simulink model "BLEMeshDiscreteEventSimulationModel"  (R2021a)
settings: Solver=VariableStepDiscrete  StartTime=0.0  StopTime=3  MaxStep=inf  RelTol=1e-3
PostLoadFcn:
  | load('bleMeshBusObjects.mat');
  | load('bleMeshDESNodePositions.mat');
  | ModelName = bdroot;
  | helperBLEMeshAssignNodeIDs(ModelName);
  | NumberOfNodes = numel(helperBLEMeshGetNodeNamesList(ModelName));
  | % Statistics
  | opcode = 0; % For creating the table
  | helperBLEMeshUpdateStatistics(opcode);
  | meshNetworkGraph = helperBLEMeshVisualizeNetwork();
InitFcn:
  | load('bleMeshBusObjects.mat');
  | load('bleMeshDESNodePositions.mat');
  | ModelName = bdroot;
  | helperBLEMeshAssignNodeIDs(ModelName);
  | NumberOfNodes = numel(helperBLEMeshGetNodeNamesList(ModelName));
  | % Statistics
  | opcode = 0; % For creating the table
  | helperBLEMeshUpdateStatistics(opcode);
  | meshNetworkGraph = helperBLEMeshVisualizeNetwork();
  | rng('default');
StartFcn:
  | if enableVisualization == 1
  | meshNetworkGraph.createNetwork();
  | end
StopFcn:
  | % Sort statisticsAtEachNode table
  | list = statisticsAtEachNode.Properties.RowNames;
  | nodeNum = cellfun(@(x)sscanf(x,'Node%d'), list);
  | [~,sortIdx] = sort(nodeNum);
  | statisticsAtEachNode = statisticsAtEachNode(sortIdx, :);
  | 
  | % Fill node statisticsAtEachNode in a cell array as input to visualization object
  | nodeStatistics = cell(1, NumberOfNodes);
  | for idx = 1:NumberOfNodes
  |     stats = {
  |         'Node Type', statisticsAtEachNode{idx, 'NodeType'}, ...
  |         'PHYTransmittedSignals', statisticsAtEachNode{idx, 'PHYTransmittedSignals'}, ...
  |         'PHYReceivedSignals', statisticsAtEachNode{idx, 'PHYReceivedSignals'}, ...
  |         'TotalCollisions', statisticsAtEachNode{idx, 'TotalCollisions'}, ...
  |         'LinkLayerTransmittedMsgs', statisticsAtEachNode{idx, 'LinkLayerTransmittedMsgs'}, ...
  |         'LinkLayerReceivedMsgs', statisticsAtEachNode{idx, 'LinkLayerReceivedMsgs'}, ...
  |         'CRCFailedMsgs', statisticsAtEachNode{idx, 'CRCFailedMsgs'}, ...
  |         'NetworkLayerTransmittedMsgs', statisticsAtEachNode{idx, 'NetworkLayerTransmittedMsgs'}, ...
  |         'NetworkLayerReceivedMsgs', statisticsAtEachNode{idx, 'NetworkLayerReceivedMsgs'}, ...
  |         'ReceivedApplicationMsgs', statisticsAtEachNode{idx, 'ReceivedApplicationMsgs'}, ...
  |         'NetworkLayerRelayedMsgs', statisticsAtEachNode{idx, 'NetworkLayerRelayedMsgs'}, ...
  |         'NetworkLayerDroppedMsgs', statisticsAtEachNode{idx, 'NetworkLayerDroppedMsgs'}};
  |     nodeStatistics{idx} = stats;
  | end
  | % Update statisticsAtEachNode in visualization object
  | if enableVisualization == 1
  | meshNetworkGraph.updateNodeStatistics(nodeStatistics);
  | end
  | % Calculate PDR of network
  | PDR = sum(statisticsAtEachNode.ReceivedApplicationMsgs) / sum(statisticsAtEachNode.NetworkLayerTransmittedMsgs);
  | fprintf('Network PDR is: %f\n', round(PDR, 4));
values from neighbouring files (symbols this model uses):
  bleMeshDESNodePositions = [0 2 4 6 8 10 12 14 16 18 20 22 ... (300 elements, 100x3)]    [bleMeshDESNodePositions.mat]    (also in bleMeshDESNodePositions19.mat = [5.030833333 8.024583333 13.395 16.32708333 22.90125 22.9012; bleMeshDESNodePositions38.mat = [2.7 5.45 5.825 10.65 13.5 13.875 18.65 21.4 18.55 2.7 5.45 ; bleMeshDESNodePositions51.mat = [2.45 5.4 2.45 5.4 5.75 10.375 13.3 10.375 13.3 13.75 18.75 ; bleMeshDESNodePositions68.mat = [0 2 4 6 8 10 12 14 16 18 0 2 ... (300 elements, 100x3)])
undefined symbols (not defined in the file or in its folder): m
libraries: BLEMeshLib x10
PostSaveFcn:
  | load('bleMeshBusObjects.mat');
  | load('bleMeshDESNodePositions.mat');
  | ModelName = bdroot;
  | helperBLEMeshAssignNodeIDs(ModelName);
  | NumberOfNodes = numel(helperBLEMeshGetNodeNamesList(ModelName));
  | % Statistics
  | opcode = 0; % For creating the table
  | helperBLEMeshUpdateStatistics(opcode);
  | meshNetworkGraph = helperBLEMeshVisualizeNetwork();
settings Model: Creator=The MathWorks, Inc.  LastModifiedBy=qcnguyen
settings SolverCC: AlgebraicLoopSolver=TrustRegion
settings DebuggingCC: SFMachineParentedDataDiag=warning

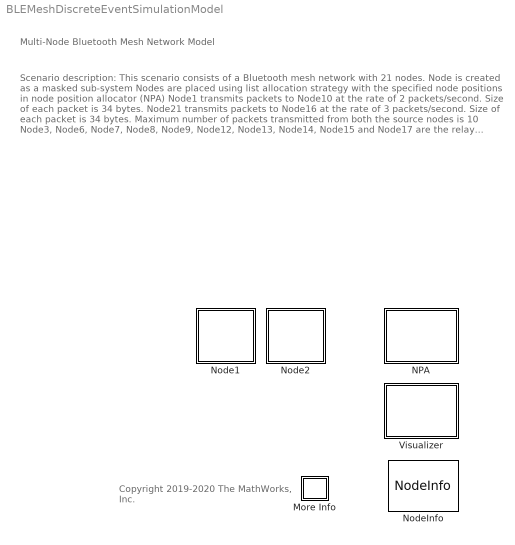
== system BLEMeshDiscreteEventSimulationModel ==
  note: Copyright 2019-2020 The MathWorks, Inc.
  note: Multi-Node Bluetooth Mesh Network Model
  note: Scenario description:
      | This scenario consists of a Bluetooth mesh network with 21 nodes. Node is created as a masked sub-system
      | Nodes are placed using list allocation strategy with the specified node positions in node position allocator (NPA)
      | Node1 transmits packets to Node10 at the rate of 2 packets/second. Size of each packet is 34 bytes.
      | Node21 transmits packets to Node16 at the rate of 3 packets/second. Size of each packet is 34 bytes.
      | Maximum number of packets transmitted from both the source nodes is 10
      | Node3, Node6, Node7, Node8, Node9, Node12, Node13, Node14, Node15 and Node17 are the relay nodes
      | Simulation time is set to 3 seconds
      | Each node contains:
      | Bluetooth mesh packet generator and receiver (mesh packet includes model, access and transport layer encoding and decoding)
      | Bluetooth mesh network layer
      | BLE link layer
      | BLE PHY Tx and Rx including interference modeling
      | Channel model
      | Nodes communicate using shared channel
      | NPA sets location of all the nodes at the start of simulation
      | Visualizer block visualizes the mesh network scenario
  More Info : Subsystem
      settings: OpenFcn=showExample('bluetooth/BLEMeshDiscreteEventSimulationExample')
      mask Display: disp('?')
  NPA : Subsystem  Tag=a  Priority=100  mask(NPA){numOfNodes=NumberOfNodes, allocationType=List Position Allocation, delta=25, direction=X, initX=0, initY=0, GridDeltaX=3, GridDeltaY=3, GridWidth=10, listName=bleMeshDESNodePositions}
      mask prompts: numOfNodes "Number of nodes:"; allocationType "Type of position allocation:"; initX "Initial X:"; initY "Initial Y:"; GridDeltaX "Delta X:"; GridDeltaY "Delta Y:"; GridWidth "Width:"; listName "Node positions:"
      mask help:
      | This block allocates node positions using three different allocation strategies –
      |
      | Linear position allocation: Places nodes uniformly in a vertical or a horizontal straight line.
      |
      | Grid position allocation: Places nodes in a grid specified by the grid properties. These properties include - direction to assign node position in the grid, initial X-Y coordinates denoting the starting location of grid, spacing in X and Y direction between successive nodes, and the number of nodes placed in a vertical or a horizontal line.
      |
      | List position allocation: Places nodes specified by a list. The list is in the form of a N-by-3 matrix, where N represents the total number of nodes and each row vector of the matrix denotes the x, y, and z coordinates of a node.
      |
      | Each of the above node position allocation strategy follows this format to specify the name of each node – <Node><n>. For example, in a network consisting of two nodes, the names of nodes can be (Node1, Node2) or (Node2, Node1).
      mask init:
      | % Visualization object
      | coder.extrinsic('assignin', 'evalin');
      | meshNetworkGraph = evalin('base', 'meshNetworkGraph');
      | 
      | % Get initial node positions by calling node position allocation strategies
      | positions = zeros(numOfNodes, 3);
      | 
      | % Linear allocation
      | if (allocationType == 1)
      |     % Allocate positions in a line with constant distance between nodes.
      |     count = 0;
      |     for i = 1:numOfNodes
      |         switch(direction)
      |             % Allocate positions in a horizontal line
      |             case 1
      |                 positions(i, 1) = initX+ delta*count;
      |                 positions(i, 2) = initY;
      |                 positions(i, 3) = 0;
      |                 % Allocate positions in a vertical line
      |             case 2
      |                 positions(i, 1) = initX;
      |                 positions(i, 2) = initY+ delta*count;
      |                 positions(i, 3)= 0;
      |         end
      |         count = count + 1;
      |     end
      |     
      | % Grid allocation 
      | elseif (allocationType == 2)
      |     for i = 1:(numOfNodes)
      |         switch(direction)
      |             case 1 % Arrange nodes row by row
      |                 positions(i, 1) = initX + GridDeltaX*(mod(i-1, GridWidth));
      |                 positions(i, 2) = initY + GridDeltaY*(floor((i-1)/GridWidth));
      |                 positions(i, 3) = 0;
      |             case 2 % Arrange nodes column by column
      |                 positions(i, 1) = initX + GridDeltaX*(floor(i-1/GridWidth));
      |                 positions(i, 2) = initY + GridDeltaY*(mod(i-1, GridWidth));
      |                 positions(i, 3) = 0;
      |         end
      |     end
      |         
      | % List allocation    
      | elseif (allocationType == 3)
      |     % Allocates node positions from a list specified by the user.
      |     positions = listName(1:(numOfNodes), :, :);
      | end
      | 
      | % Set the positions of nodes
      | for i = 1:numOfNodes
      |     % Get the block which contains matching node id as a parameter
      |     blockName = find_system(bdroot,'NodeID',num2str(i));
      |     posID = str2num(blockName{1}(strlength([bdroot '/Node'])+1:end));
      |     try
      |         % Convert position from number to string
      |         b = num2str(['[' [num2str(positions(posID, :)) ']']]);
      |         % Assign new position to a node subsystem
      |         set_param(blockName{1},'NodePosition', b);
      |     catch
      |     end
      | end
      | 
      | positions = positions(:,1:2);
      | 
      | % Update configuration
      | meshNetworkGraph.NumberOfNodes = numOfNodes;
      | meshNetworkGraph.NodePositionType = 'UserInput';
      | meshNetworkGraph.Positions = positions;
      | %meshNetworkGraph.VicinityRange = 25;
      | meshNetworkGraph.Title = 'Bluetooth Mesh Network';
      | 
      | assignin('base', 'meshNetworkGraph', meshNetworkGraph);
      mask TypeOptions allocationType: Linear Position Allocation | Grid Position Allocation | List Position Allocation
      mask Callback allocationType:
      | % Get allocation type selected by user
      | maskStr = get_param(gcb,'allocationType');
      | % Set mask parameters visibilities based on allocation type
      | if strcmp(maskStr,'Linear Position Allocation')
      |     set_param(gcb,'MaskVisibilities',{'on','on','on','on','on','on','off','off','off','off'});
      | elseif strcmp(maskStr,'List Position Allocation')
      |     set_param(gcb,'MaskVisibilities',{'on','on','off','off','off','off','off','off','off','on'});
      | elseif strcmp(maskStr,'Grid Position Allocation')
      |     set_param(gcb,'MaskVisibilities',{'on','on','off','on','on','on','on','on','on','off'});
      | end
      | % Clear variables
      | clear maskStr;
      mask TypeOptions direction: X | Y
      mask Display: disp('NPA');
  Node1 : Subsystem  mask{NodePosition=[2.45        1.65           0], NodeID=1}
      mask prompts: NodePosition "Node position:"; NodeID "Node id:"
      mask init:
      | global NodeInfo
      | ElementAddress = hex2dec(reshape(dec2hex(NodeID, 4), 2, [])');
      | NodeInfo(NodeID).NodeID = NodeID;
      | NodeInfo(NodeID).ElementAddress = ElementAddress;
      mask DialogControl DescGroupVar Prompt: Bluetooth device
      mask DialogControl DescTextVar Prompt: Bluetooth mesh device communicates over GAP bearer including:  Application layer, Network layer, Link layer and Physical layer
      mask Display: disp(['Bluetooth' newline 'Node']);
  Node2 : Subsystem  mask{NodePosition=[5.4        1.65           0], NodeID=2}
      mask prompts: NodePosition "Node position:"; NodeID "Node id:"
      mask init:
      | global NodeInfo
      | ElementAddress = hex2dec(reshape(dec2hex(NodeID, 4), 2, [])');
      | NodeInfo(NodeID).NodeID = NodeID;
      | NodeInfo(NodeID).ElementAddress = ElementAddress;
      mask DialogControl DescGroupVar Prompt: Bluetooth device
      mask DialogControl DescTextVar Prompt: Bluetooth mesh device communicates over GAP bearer including:  Application layer, Network layer, Link layer and Physical layer
      mask Display: disp(['Bluetooth' newline 'Node']);
  NodeInfo : DataStoreMemory  DataStoreName=NodeInfo  ReadBeforeWriteMsg=warning  WriteAfterWriteMsg=warning  WriteAfterReadMsg=warning  ShowAdditionalParam=off  OutDataTypeStr=Bus: NodeInfo  Dimensions=NumberOfNodes
      mask DialogControl DescGroupVar Prompt: NodeInfo
      mask DialogControl DescTextVar Prompt: This block is used to store and share node-related information such as NodeID and ElementAddress. There are no configuration options for this block.
  Visualizer : Subsystem  Tag=a  Priority=100  mask(Subsystem){enableVisualization=on}
      mask prompts: enableVisualization "Enable Visualization"
      mask init:
      | % Skip codegen
      | coder.extrinsic('assignin', 'evalin', 'get_param');
      | assignin('base', 'enableVisualization', enableVisualization);
      | % If visualization is enabled update the configuration in visualization
      | % object
      | if (enableVisualization == 1)
      |     meshNetworkGraph = evalin('base', 'meshNetworkGraph');
      |     NumberOfNodes = evalin('base', 'NumberOfNodes');
      |     % Get srcDstPairs and relayNodes from assigned configuration
      |     srcDstPairs = zeros(1, 0);
      |     relayNodes = zeros(1, 0);
      |     srcDstPairsIdx = 1;
      |     relayIdx = 1;
      |     for i = 1:NumberOfNodes
      |         appState = get_param([bdroot '/Node' num2str(i) '/AppDES'], 'ApplicationState');
      |         if strcmp(appState, '0') == false
      |             destName = get_param([bdroot '/Node' num2str(i) '/AppDES'], 'DestinationNode');
      |             %str = split(destName, 'e');
      |             srcDstPairs(srcDstPairsIdx, 1) = i;
      |             srcDstPairs(srcDstPairsIdx, 2) = str2double(destName);
      |             %srcDstPairs(srcDstPairsIdx, 2) = str2double(str{2});
      |             srcDstPairsIdx = srcDstPairsIdx + 1;
      |         end
      |         relay = get_param([bdroot '/Node' num2str(i) '/Network layer'], 'Relay');
      |         if strcmp(relay, 'Off') == false
      |             relayNodes(relayIdx) = i;
      |             relayIdx = relayIdx + 1;
      |         end
      |     end
      |     meshNetworkGraph.NumberOfNodes = NumberOfNodes;
      |     meshNetworkGraph.SrcDstPairs = srcDstPairs;
      |     nodeStates = zeros(1, NumberOfNodes);
      |     for i=1:NumberOfNodes
      |         % Relay node
      |         if any(i == relayNodes)
      |             nodeStates(i) = 2;
      |             % End node
      |         else
      |             nodeStates(i) = 1;
      |         end
      |     end
      |     meshNetworkGraph.NodeState = nodeStates;
      |     meshNetworkGraph.DisplayProgressBar = false;
      |     assignin('base', 'meshNetworkGraph', meshNetworkGraph);
      | end
      mask DialogControl DescGroupVar Prompt: Visualizer
      mask DialogControl DescTextVar Prompt: Visualizes Bluetooth mesh network based on the given configuration
      mask Display: disp('Visualizer');

== system BLEMeshDiscreteEventSimulationModel/More Info ==

== system BLEMeshDiscreteEventSimulationModel/NPA ==

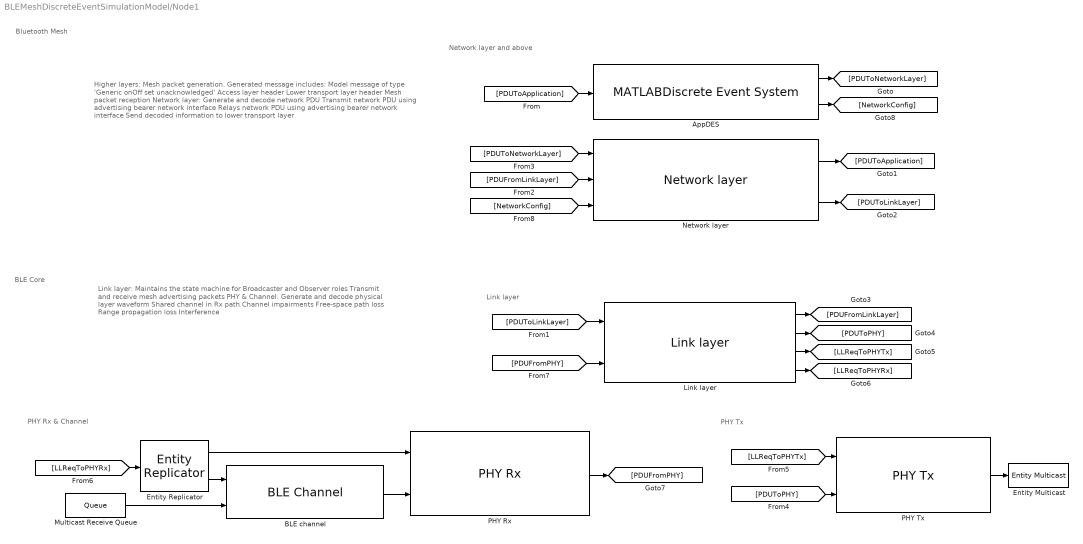
== system BLEMeshDiscreteEventSimulationModel/Node1 ==
  note: Network layer and above
  note: Link layer
  note: Link layer:
      | Maintains the state machine for Broadcaster and Observer roles
      | Transmit and receive mesh advertising packets
      |
      | PHY & Channel:
      | Generate and decode physical layer waveform
      | Shared channel in Rx path
      | Channel impairments
      | Free-space path loss
      | Range propagation loss
      | Interference
  note: BLE Core
  note: Bluetooth Mesh
  note: PHY Rx & Channel
  note: PHY Tx
  note: Higher layers:
      | Mesh packet generation. Generated message includes:
      | Model message of type 'Generic onOff set unacknowledged'
      | Access layer header
      | Lower transport layer header
      | Mesh packet reception
      |
      | Network layer:
      | Generate and decode network PDU
      | Transmit network PDU using advertising bearer network interface
      | Relays network PDU using advertising bearer network interface
      | Send decoded information to lower transport layer
  AppDES : MATLABDiscreteEventSystem  InputPortMessageModes=m  OutputPortMessageModes=m,m  System=AppDES  NodeID=1  DestinationNode=1  ApplicationState=0  TTL=127  SourceRate=1  TotalPackets=1  SimulateUsing=Code generation
      mask Type: AppDES
      mask Display:
      | disp('AppDES');
      | port_label('input',1,'transportPDUIn');
      | port_label('output',1,'transportPDUOut');
      | port_label('output',2,'networkConfig');
  BLE channel : BLEMeshLib/BLE Channel  RangePropagationLoss=On  FSPLModel=On  RxRange=7  NodePosition=NodePosition  NodeID=NodeID  SimulateUsing=Code generation
  Entity Multicast : EntityMulticast  InputPortMessageModes=m  MulticastTag=channel
  Entity Replicator : EntityReplicator  InputPortMessageModes=m  OutputPortMessageModes=m,m
  Link layer : BLEMeshLib/Link layer  RandomAdvertising=On  AdvertisingInterval=20  ScanInterval=30  NodeID=NodeID  SimulateUsing=Code generation  mask(helperBLEMeshLinkLayerDES){}
  Multicast Receive Queue : Queue  OutputPortMessageModes=m  EntityArrivalSource=Multicast  MulticastTag=channel
  Network layer : BLEMeshLib/Network layer  Relay=Off  ElementAddresses=ElementAddress  NetworkTransmitCount=3  NetworkTransmitInterval=30  RelayRetransmitCount=3  RelayRetransmitInterval=30  NodeID=NodeID  SimulateUsing=Code generation
  PHY Rx : BLEMeshLib/PHY Rx  NoiseFigure=0  NodeID=NodeID  SimulateUsing=Interpreted execution
  PHY Tx : BLEMeshLib/PHY Tx  TxPower=0  NodePosition=NodePosition  NodeID=NodeID  SimulateUsing=Interpreted execution
  wires:
  Link layer/4 -> [LLReqToPHYRx]
  Link layer/2 -> [PDUToPHY]
  Link layer/3 -> [LLReqToPHYTx]
  Link layer/1 -> [PDUFromLinkLayer]
  [PDUToNetworkLayer] -> Network layer/1
  Network layer/1 -> [PDUToApplication]
  [PDUFromLinkLayer] -> Network layer/2
  Entity Replicator/1 -> PHY Rx/1
  PHY Rx/1 -> [PDUFromPHY]
  BLE channel/1 -> PHY Rx/2
  PHY Tx/1 -> Entity Multicast/1
  [LLReqToPHYRx] -> Entity Replicator/1
  Multicast Receive Queue/1 -> BLE channel/2
  Entity Replicator/2 -> BLE channel/1
  [LLReqToPHYTx] -> PHY Tx/1
  [PDUToPHY] -> PHY Tx/2
  Network layer/2 -> [PDUToLinkLayer]
  [PDUToLinkLayer] -> Link layer/1
  [PDUFromPHY] -> Link layer/2
  AppDES/1 -> [PDUToNetworkLayer]
  [PDUToApplication] -> AppDES/1
  [NetworkConfig] -> Network layer/3
  AppDES/2 -> [NetworkConfig]

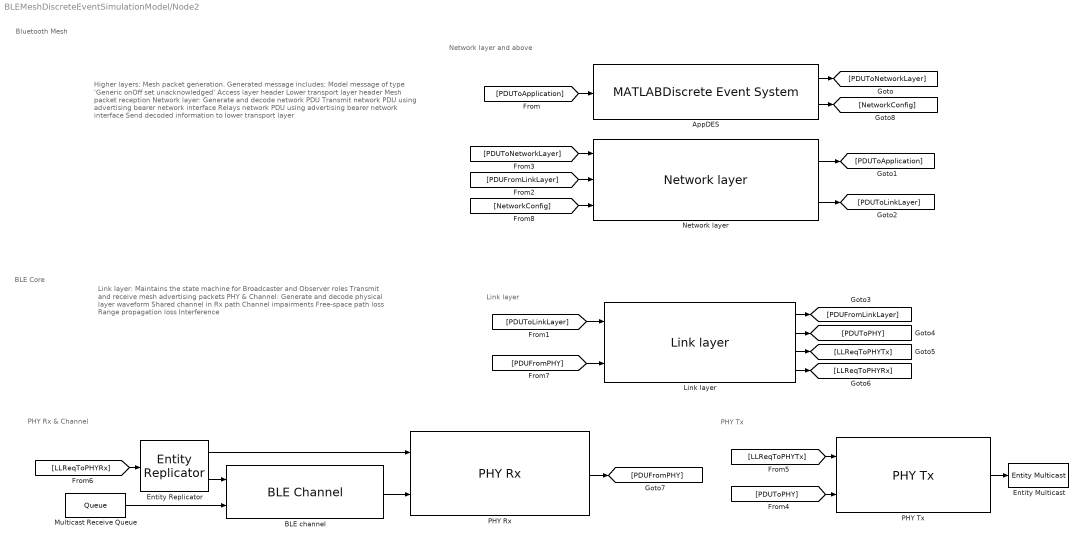
== system BLEMeshDiscreteEventSimulationModel/Node2 ==
  note: Network layer and above
  note: Link layer
  note: Link layer:
      | Maintains the state machine for Broadcaster and Observer roles
      | Transmit and receive mesh advertising packets
      |
      | PHY & Channel:
      | Generate and decode physical layer waveform
      | Shared channel in Rx path
      | Channel impairments
      | Free-space path loss
      | Range propagation loss
      | Interference
  note: BLE Core
  note: Bluetooth Mesh
  note: PHY Rx & Channel
  note: PHY Tx
  note: Higher layers:
      | Mesh packet generation. Generated message includes:
      | Model message of type 'Generic onOff set unacknowledged'
      | Access layer header
      | Lower transport layer header
      | Mesh packet reception
      |
      | Network layer:
      | Generate and decode network PDU
      | Transmit network PDU using advertising bearer network interface
      | Relays network PDU using advertising bearer network interface
      | Send decoded information to lower transport layer
  AppDES : MATLABDiscreteEventSystem  InputPortMessageModes=m  OutputPortMessageModes=m,m  System=AppDES  NodeID=2  DestinationNode=1  ApplicationState=0  TTL=127  SourceRate=1  TotalPackets=1  SimulateUsing=Code generation
      mask Type: AppDES
      mask Display:
      | disp('AppDES');
      | port_label('input',1,'transportPDUIn');
      | port_label('output',1,'transportPDUOut');
      | port_label('output',2,'networkConfig');
  BLE channel : BLEMeshLib/BLE Channel  RangePropagationLoss=On  FSPLModel=On  RxRange=6  NodePosition=NodePosition  NodeID=NodeID  SimulateUsing=Code generation
  Entity Multicast : EntityMulticast  InputPortMessageModes=m  MulticastTag=channel
  Entity Replicator : EntityReplicator  InputPortMessageModes=m  OutputPortMessageModes=m,m
  Link layer : BLEMeshLib/Link layer  RandomAdvertising=On  AdvertisingInterval=20  ScanInterval=30  NodeID=NodeID  SimulateUsing=Code generation  mask(helperBLEMeshLinkLayerDES){}
  Multicast Receive Queue : Queue  OutputPortMessageModes=m  EntityArrivalSource=Multicast  MulticastTag=channel
  Network layer : BLEMeshLib/Network layer  Relay=Off  ElementAddresses=ElementAddress  NetworkTransmitCount=3  NetworkTransmitInterval=30  RelayRetransmitCount=3  RelayRetransmitInterval=30  NodeID=NodeID  SimulateUsing=Code generation
  PHY Rx : BLEMeshLib/PHY Rx  NoiseFigure=0  NodeID=NodeID  SimulateUsing=Interpreted execution
  PHY Tx : BLEMeshLib/PHY Tx  TxPower=20  NodePosition=NodePosition  NodeID=NodeID  SimulateUsing=Interpreted execution
  wires:
  Link layer/4 -> [LLReqToPHYRx]
  Link layer/2 -> [PDUToPHY]
  Link layer/3 -> [LLReqToPHYTx]
  Link layer/1 -> [PDUFromLinkLayer]
  [PDUToNetworkLayer] -> Network layer/1
  Network layer/1 -> [PDUToApplication]
  [PDUFromLinkLayer] -> Network layer/2
  Entity Replicator/1 -> PHY Rx/1
  PHY Rx/1 -> [PDUFromPHY]
  BLE channel/1 -> PHY Rx/2
  PHY Tx/1 -> Entity Multicast/1
  [LLReqToPHYRx] -> Entity Replicator/1
  Multicast Receive Queue/1 -> BLE channel/2
  Entity Replicator/2 -> BLE channel/1
  [LLReqToPHYTx] -> PHY Tx/1
  [PDUToPHY] -> PHY Tx/2
  Network layer/2 -> [PDUToLinkLayer]
  [PDUToLinkLayer] -> Link layer/1
  [PDUFromPHY] -> Link layer/2
  AppDES/1 -> [PDUToNetworkLayer]
  [PDUToApplication] -> AppDES/1
  [NetworkConfig] -> Network layer/3
  AppDES/2 -> [NetworkConfig]

== system BLEMeshDiscreteEventSimulationModel/Visualizer ==
